simulink model "FTG"  (R2022a)
settings: Solver=ode4  StartTime=0.0  StopTime=100  FixedStep=0.01  RelTol=1e-3
PreLoadFcn:
  | listing = dir;
  | if (contains([listing .name], 'FLCC')) && (contains([listing .name], 'DYN'))
  |     addpath('./DYN', './FLCC', './FTG', './GPS', './INS', './MAP', './RALT', './TCAF');
  | elseif (contains([listing .name], 'FTG.slx'))
  |     addpath('../DYN', '../FLCC', '../FTG', '../GPS', '../INS', '../MAP', '../RALT', '../TCAF');
  | else
  | 
  | end
  | 
  | load('BUS_STRUCTURE_DYN.mat');
  | load('BUS_STRUCTURE_FLCC.mat');
  | load('BUS_STRUCTURE_RALT.mat');
  | load('BUS_STRUCTURE_INS.mat');
  | load('BUS_STRUCTURE_GPS.mat');
  | load('BUS_STRUCTURE_SENSOR_INPUT.mat');
  | load('BusStructureDTF.mat');
  | load('BusStructureGCAWS.mat');
  | FTG_initState;
  | 
  | % Random number seed
  | if ~exist('ranNumSeed', 'var')
  |     ranNumSeed = 2034;
  | end
InitFcn:
  | listing = dir;
  | if (contains([listing .name], 'FLCC')) && (contains([listing .name], 'DYN'))
  |     addpath('./DYN', './FLCC', './FTG', './GPS', './INS', './MAP', './RALT', './TCAF');
  | elseif (contains([listing .name], 'FTG.slx'))
  |     addpath('../DYN', '../FLCC', '../FTG', '../GPS', '../INS', '../MAP', '../RALT', '../TCAF');
  | else
  | 
  | end
  | 
  | load('BUS_STRUCTURE_DYN.mat');
  | load('BUS_STRUCTURE_FLCC.mat');
  | load('BUS_STRUCTURE_RALT.mat');
  | load('BUS_STRUCTURE_INS.mat');
  | load('BUS_STRUCTURE_GPS.mat');
  | load('BUS_STRUCTURE_SENSOR_INPUT.mat');
  | load('BusStructureDTF.mat');
  | load('BusStructureGCAWS.mat');
  | FTG_initState;
  | 
  | % Random number seed
  | if ~exist('ranNumSeed', 'var')
  |     ranNumSeed = 2034;
  | end
values from neighbouring files (symbols this model uses):
  initState = struct    [FTG_initState.m]
undefined symbols (not defined in the file or in its folder): GPS, INS, RALT
libraries: simulink_extras x8
settings Model: Creator=ASCL  LastModifiedBy=ASCL
settings DataIOCC: ExternalInput=FTGScenario.getElement('IN_STICK'), [], [],FTGScenario.getElement('IN_FLIGHT_CMD'), []  LoadExternalInput=on  SaveOutput=off  DSMLogging=off  SaveTime=off  ReturnWorkspaceOutputs=off
settings OptimizationCC: BlockReduction=off  DefaultParameterBehavior=Inlined  UseDivisionForNetSlopeComputation=on  GainParamInheritBuiltInType=on  UseFloatMulNetSlope=on  ExpressionFolding=off  PassReuseOutputArgsAs=Individual arguments  ZeroExternalMemoryAtStartup=off  ZeroInternalMemoryAtStartup=off  EfficientFloat2IntCast=on  LifeSpan=inf  OptimizeBlockOrder=speed  DifferentSizesBufferReuse=on  EfficientTunableParamExpr=on
settings DebuggingCC: SignalInfNanChecking=warning  ReadBeforeWriteMsg=EnableAllAsError  WriteAfterWriteMsg=EnableAllAsError  WriteAfterReadMsg=EnableAllAsError  IntegerOverflowMsg=error  ParameterTunabilityLossMsg=error  UniqueDataStoreMsg=error  AssertControl=DisableAll  NonBusSignalsTreatedAsBus=error  SFInvalidInputDataAccessInChartInitDiag=error  SFTransitionOutsideNaturalParentDiag=error  SFUnreachableExecutionPathDiag=error  SFUndirectedBroadcastEventsDiag=error  IntegerSaturationMsg=error
settings HardwareCC: ProdBitPerPointer=32  ProdBitPerSizeT=32  ProdBitPerPtrDiffT=32  ProdLargestAtomicInteger=Long  ProdLargestAtomicFloat=Double  ProdEndianess=BigEndian  ProdWordSize=32  ProdLongLongMode=on  ProdHWDeviceType=Freescale->MPC83xx
settings ModelReferenceCC: ModelReferenceNumInstancesAllowed=Single
settings SFSimCC: SimCustomHeaderCode="#include \"MAP.h\""  SimUserSources=MAP.c  SimUserLibraries=WS2_32.LIB  CompileTimeRecursionLimit=0  EnableRuntimeRecursion=off  MATLABDynamicMemAlloc=off
settings RTWCC: SystemTargetFile=ert.tlc  TemplateMakefile=ert_default_tmf  GenerateReport=on  RTWUseSimCustomCode=on  CustomHeaderCode="#include \"MAP.h\""  CustomSource=MAP.c  CustomLibrary=WS2_32.LIB  BuildConfiguration=Faster Runs  IncludeHyperlinkInReport=on  LaunchReport=on  GenerateTraceInfo=on  GenerateTraceReport=on  GenerateTraceReportSl=on  GenerateTraceReportSf=on  GenerateTraceReportEml=on  GenerateCodeMetricsReport=on
settings CodeAppCC: ForceParamTrailComments=on  IgnoreCustomStorageClasses=off  OperatorAnnotations=on  SimulinkDataObjDesc=on  SFDataObjDesc=on  MATLABFcnDesc=on  InsertBlockDesc=on  StateflowObjectComments=on  MATLABSourceComments=on  EnableCustomComments=on  InlinedPrmAccess=Macros  ReqsInCode=on
settings ERTTargetCC: TargetLangStandard=C99 (ISO)  UtilityFuncGeneration=Shared location  GenerateSampleERTMain=on  IncludeMdlTerminateFcn=off  CombineSignalStateStructs=on  SupportAbsoluteTime=off  SupportNonFinite=off  SupportVariableSizeSignals=on  ParenthesesLevel=Standards  CastingMode=Standards  GenerateSharedConstants=off  InlinedParameterPlacement=NonHierarchical  ERTCustomFileTemplate=example_file_process.tlc  RateTransitionBlockCode=Function  PreserveIfCondition=on  ConvertIfToSwitch=off  EnableSignedLeftShifts=off  EnableSignedRightShifts=off

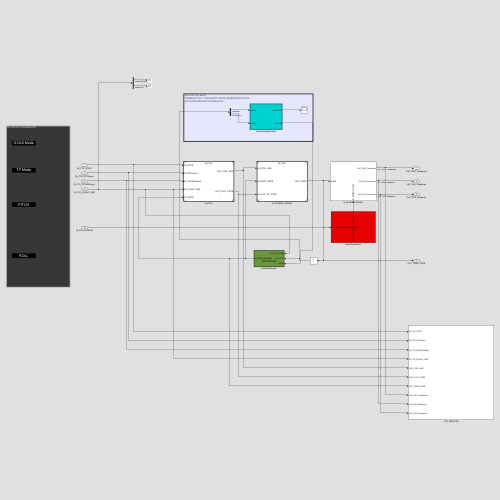
[thumbnail: Simulink's stored preview of the top-level diagram]
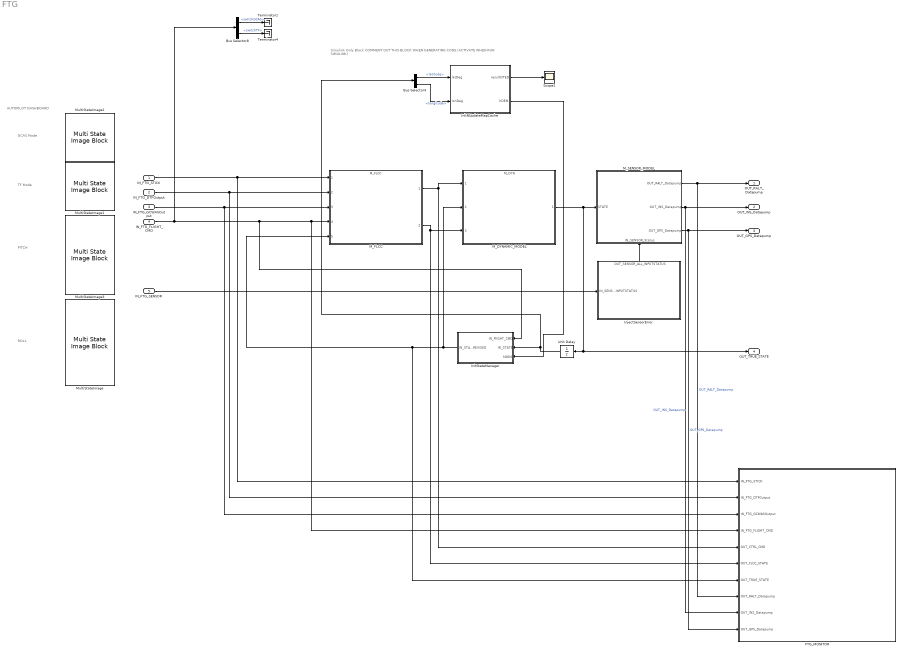
== system FTG ==
  note: GCAS Mode
  note: TF Mode
  note: AUTOPILOT DASHBOARD
  note: ROLL
  note: Simulink Only Block
      | COMMENT OUT THIS BLOCK WHEN GENERATING CODE
      | (ACTIVATE WHEN RUN SIMULINK)
  note: PITCH
  IN_FTG_STICK : Inport  OutDataTypeStr=Bus: BUS_FLCC_STICK  Interpolate=off  BusOutputAsStruct=on
  IN_FTG_DTFOutput : Inport  Port=2  OutDataTypeStr=Bus: DTFOutput  Interpolate=off  BusOutputAsStruct=on
  IN_FTG_GCWASOutput : Inport  Port=3  OutDataTypeStr=Bus: GCAWSOutput  Interpolate=off  BusOutputAsStruct=on
  IN_FTG_FLIGHT_CMD : Inport  Port=4  OutDataTypeStr=Bus: BUS_FLCC_FLIGHT_CMD  Interpolate=off  BusOutputAsStruct=on
  IN_FTG_SENSOR : Inport  Port=5  OutDataTypeStr=Bus: BUS_SENSOR_ALL_INPUTSTATUS  Interpolate=off  BusOutputAsStruct=on
  Bus Selector4 : BusSelector  OutputSignals=latitude,longitude
  Bus Selector8 : BusSelector  OutputSignals=switchGCAS,switchTF
  FTG_MONITOR : Subsystem
  InitNUpdateMapCache : Subsystem  TreatAsAtomicUnit=on
  InitStateManager : MATLAB Function  TreatAsAtomicUnit=on  SystemSampleTime=0.01
  InjectSensorError : Subsystem
      settings: PortSchema="{\"entries\":[{\"content\":{\"sides\":[{\"content\":{\"connectorIds\":[]},\"type\":\"ConnectorPlacement.EquallySpacedRectSide\",\"uuid\":\"6514be54-5250-42b1-89ec-96b3ca3204a4\"},{\"content\":{\"connectorIds\":[\"Out1\"],\"side\":\"RIGHT\"},\"type\":\"ConnectorPlacement.EquallySpacedRectSide\",\"uuid\":\"5a471b5b-ecab-4b12-91ae-851436c3af59\"},{\"content\":{\"connectorIds\":[\"In1\"],\"side\":\"TOP\"},\"type\":\"ConnectorPlacement.EquallySpacedRectSide\",\"uuid\":\"7b7a7584-bd38-4309-866b-d1039bf73b0c\"}]},\"type\":\"ConnectorPlacement.EquallySpacedConnector\",\"uuid\":\"354782b0-b839-451e-ba58-c4baa2a23659\"}],\"packageUris\":[\"http://schema.mathworks.com/mf0/Connector/R2020b\"],\"version\":\"1.0\"}"
  M_DYNAMIC_MODEL : ModelReference  ModelNameDialog=M_DYN.slx  SimulationMode=Normal  ModelReferenceVersion=1.350
  M_FLCC : ModelReference  ModelNameDialog=M_FLCC.slx  SimulationMode=Normal  ModelReferenceVersion=1.2865
  M_SENSOR_MODEL : Subsystem
      settings: PortSchema="{\"entries\":[{\"content\":{\"sides\":[{\"content\":{\"connectorIds\":[\"In1\"]},\"type\":\"ConnectorPlacement.EquallySpacedRectSide\",\"uuid\":\"880db95d-6046-467e-9f42-4d7f31e7d636\"},{\"content\":{\"connectorIds\":[\"Out1\",\"Out2\",\"Out3\"],\"side\":\"RIGHT\"},\"type\":\"ConnectorPlacement.EquallySpacedRectSide\",\"uuid\":\"4b6edf19-899b-47c2-bce1-8d6f85bc3049\"},{\"content\":{\"connectorIds\":[],\"side\":\"TOP\"},\"type\":\"ConnectorPlacement.EquallySpacedRectSide\",\"uuid\":\"fbda278b-8c92-4691-b142-226c9beb0c5e\"},{\"content\":{\"connectorIds\":[\"In2\"],\"side\":\"BOTTOM\"},\"type\":\"ConnectorPlacement.EquallySpacedRectSide\",\"uuid\":\"c82397e7-e882-4f57-bc38-1d7b6d57b901\"}]},\"type\":\"ConnectorPlacement.EquallySpacedConnector\",\"uuid\":\"2b9ff209-30b8-444e-97ac-554833487782\"}],\"packageUris\":[\"http://schema.mathworks.com/mf0/Connector/R2020b\"],\"version\":\"1.0\"}"
  MultiStateImage{,1..3} (4 alike) : MultiStateImageBlock
  Scope1 : Scope
  Terminator1 : Terminator
  Terminator4 : Terminator
  Unit Delay : UnitDelay  InitialCondition=initState  SampleTime=0.01  HasFrameUpgradeWarning=on
  OUT_RALT_Datapump : Outport  OutDataTypeStr=Bus: BUS_SENSOR_RALT_DP  SampleTime=0.01  BusOutputAsStruct=on
  OUT_INS_Datapump : Outport  Port=2  OutDataTypeStr=Bus: BUS_SENSOR_INS_DP  SampleTime=0.01  BusOutputAsStruct=on
  OUT_GPS_Datapump : Outport  Port=3  OutDataTypeStr=Bus: BUS_SENSOR_GPS_DP  SampleTime=0.01  BusOutputAsStruct=on
  OUT_TRUE_STATE : Outport  Port=4  OutDataTypeStr=Bus: BUS_DYN_STATE  SampleTime=0.01  BusOutputAsStruct=on
  wires:
  Bus Selector4/2 -> InitNUpdateMapCache/2(lonDeg)  "<longitude>"
  M_FLCC/2 -> M_DYNAMIC_MODEL/3, FTG_MONITOR/6(OUT_FLCC_STATE)
  IN_FTG_GCWASOutput/1 -> FTG_MONITOR/3(IN_FTG_GCWASOutput), M_FLCC/3
  M_SENSOR_MODEL/1(OUT_RALT_Datapump) -> OUT_RALT_Datapump/1, FTG_MONITOR/8(OUT_RALT_Datapump)  "OUT_RALT_Datapump"
  M_SENSOR_MODEL/3(OUT_GPS_Datapump) -> OUT_GPS_Datapump/1, FTG_MONITOR/10(OUT_GPS_Datapump)  "OUT_GPS_Datapump"
  IN_FTG_STICK/1 -> FTG_MONITOR/1(IN_FTG_STICK), M_FLCC/1
  IN_FTG_DTFOutput/1 -> FTG_MONITOR/2(IN_FTG_DTFOutput), M_FLCC/2
  Bus Selector4/1 -> InitNUpdateMapCache/1(latDeg)  "<latitude>"
  M_SENSOR_MODEL/2(OUT_INS_Datapump) -> OUT_INS_Datapump/1, FTG_MONITOR/9(OUT_INS_Datapump)  "OUT_INS_Datapump"
  M_FLCC/1 -> FTG_MONITOR/5(OUT_CTRL_CMD), M_DYNAMIC_MODEL/1
  M_DYNAMIC_MODEL/1 -> Unit Delay/1, OUT_TRUE_STATE/1, M_SENSOR_MODEL/1(STATE)
  Bus Selector8/2 -> Terminator4/1  "<switchTF>"
  Bus Selector8/1 -> Terminator1/1  "<switchGCAS>"
  InitNUpdateMapCache/1(resultDTED) -> Scope1/1
  IN_FTG_SENSOR/1 -> InjectSensorError/1(IN_SENSOR_ALL_INPUTSTATUS)
  InjectSensorError/1(OUT_SENSOR_ALL_INPUTSTATUS) -> M_SENSOR_MODEL/2(IN_SENSOR_Status)
  IN_FTG_FLIGHT_CMD/1 -> InitStateManager/1(IN_FlIGHT_CMD), FTG_MONITOR/4(IN_FTG_FLIGHT_CMD), M_FLCC/4, Bus Selector8/1
  InitStateManager/1(IN_STATE_REVISED) -> M_DYNAMIC_MODEL/2, FTG_MONITOR/7(OUT_TRUE_STATE), M_FLCC/5
  Unit Delay/1 -> InitStateManager/2(IN_STATE), Bus Selector4/1
  InitNUpdateMapCache/2(hDEM) -> InitStateManager/3(hDEM)

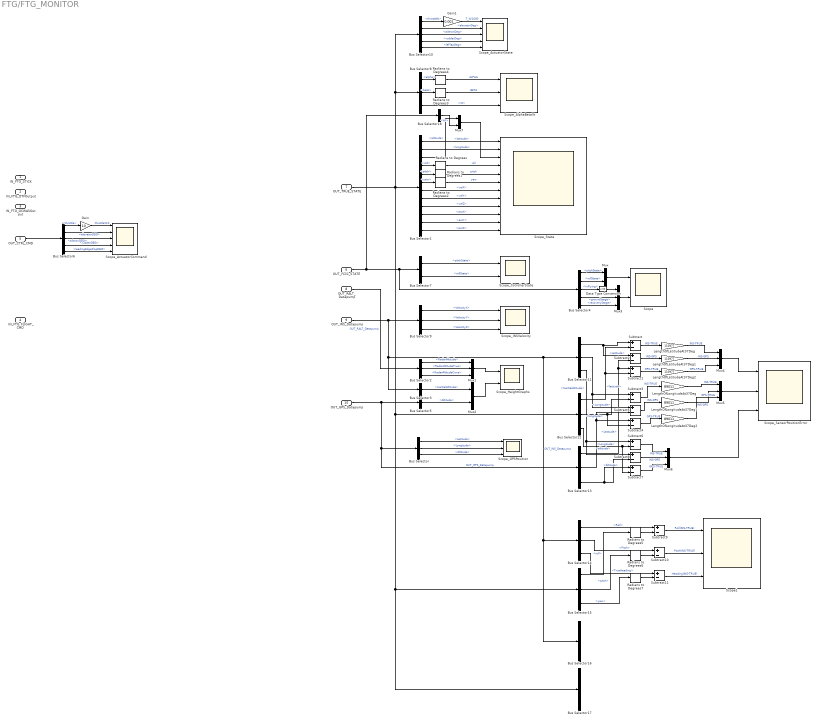
== system FTG/FTG_MONITOR ==
  IN_FTG_STICK : Inport
  IN_FTG_DTFOutput : Inport  Port=2
  IN_FTG_GCWASOutput : Inport  Port=3
  IN_FTG_FLIGHT_CMD : Inport  Port=4
  OUT_CTRL_CMD : Inport  Port=5
  OUT_FLCC_STATE : Inport  Port=6
  OUT_TRUE_STATE : Inport  Port=7
  OUT_RALT_Datapump : Inport  Port=8
  OUT_INS_Datapump : Inport  Port=9
  OUT_GPS_Datapump : Inport  Port=10
  Bus Selector : BusSelector  OutputSignals=Latitude,Longitude,Altitude
  Bus Selector1 : BusSelector  OutputSignals=latitude,longitude,altitude,roll,pitch,yaw,velX,velY,velZ,accX,accY,accZ
  Bus Selector10 : BusSelector  OutputSignals=throttleN,elevatorDeg,aileronDeg,rudderDeg,leFlapDeg
  Bus Selector11 : BusSelector  OutputSignals=Latitude,Longitude,InertialAltitude
  Bus Selector12 : BusSelector  OutputSignals=latitude,longitude,altitude
  Bus Selector13 : BusSelector  OutputSignals=Latitude,Longitude,Altitude
  Bus Selector14 : BusSelector  OutputSignals=Roll,Pitch,TrueHeading
  Bus Selector15 : BusSelector  OutputSignals=roll,pitch,yaw
  Bus Selector16 : BusSelector  OutputSignals=VelocityX,VelocityY,VelocityZ
  Bus Selector17 : BusSelector  OutputSignals=velX,velY,velZ
  Bus Selector18 : BusSelector  OutputSignals=h0
  Bus Selector2 : BusSelector  OutputSignals=RadarAltitude,RadarAltitudeTrue,RadarAltitudeCone
  Bus Selector3 : BusSelector  OutputSignals=InertialAltitude
  Bus Selector4 : BusSelector  OutputSignals=pitchState,rollState,inFlying,groundStage,recoveryStage
  Bus Selector5 : BusSelector  OutputSignals=Altitude
  Bus Selector6 : BusSelector  OutputSignals=throttle,elevatorDEG,aileronDEG,rudderDEG,leadingEdgeFlapDEG
  Bus Selector7 : BusSelector  OutputSignals=pitchState,rollState
  Bus Selector8 : BusSelector  OutputSignals=alpha,beta,Vt
  Bus Selector9 : BusSelector  OutputSignals=VelocityX,VelocityY,VelocityZ
  Data Type Conversion : DataTypeConversion  OutDataTypeStr=uint8  SaturateOnIntegerOverflow=off  RndMeth=Floor
  Gain : Gain  Gain=10
  Gain1 : Gain  Gain=0.001
  LengthOfLatitudeAt37Deg : Gain  Gain=110977
  LengthOfLatitudeAt37Deg1 : Gain  Gain=110977
  LengthOfLatitudeAt37Deg2 : Gain  Gain=110977
  LengthOfLongitudeAt37Deg : Gain  Gain=89011
  LengthOfLongitudeAt37Deg1 : Gain  Gain=89011
  LengthOfLongitudeAt37Deg2 : Gain  Gain=89011
  Mux : Mux  Inputs=2
  Mux{1,3..6} (5 alike) : Mux  Inputs=3
  Mux2 : Mux  Inputs=2
  Mux7 : Mux  Inputs=2
  Radians to Degrees{,1..7} (8 alike) : simulink_extras/Transformations/Radians to Degrees
  Scope : Scope  NumInputPorts=2
  Scope1 : Scope  NumInputPorts=3
  Scope_ActuatorCommand : Scope  NumInputPorts=5
  Scope_ActuatorState : Scope  NumInputPorts=5
  Scope_AlphaBetaVt : Scope  NumInputPorts=3
  Scope_CotrollerState : Scope  NumInputPorts=2
  Scope_GPSPosition : Scope  NumInputPorts=3
  Scope_HeightGraphs : Scope  NumInputPorts=2
  Scope_INSVelocity : Scope  NumInputPorts=3
  Scope_SensorPositionError : Scope  NumInputPorts=3
  Scope_State : Scope  NumInputPorts=12
  Subtract{,1..11} (12 alike) : Sum  Inputs=+-
  wires:
  Bus Selector1/9 -> Scope_State/9  "<velZ>"
  Bus Selector1/10 -> Scope_State/10  "<accX>"
  Bus Selector1/4 -> Radians to Degrees/1  "<roll>"
  Bus Selector1/1 -> Scope_State/1  "<latitude>"
  Radians to Degrees/1 -> Scope_State/4  "roll"
  Radians to Degrees1/1 -> Scope_State/5  "pitch"
  Bus Selector1/7 -> Scope_State/7  "<velX>"
  Bus Selector1/12 -> Scope_State/12  "<accZ>"
  Bus Selector1/2 -> Scope_State/2  "<longitude>"
  Bus Selector1/8 -> Scope_State/8  "<velY>"
  Bus Selector1/11 -> Scope_State/11  "<accY>"
  Bus Selector1/6 -> Radians to Degrees2/1  "<yaw>"
  Radians to Degrees2/1 -> Scope_State/6  "yaw"
  Bus Selector1/3 -> Mux7/1  "<altitude>"
  Bus Selector1/5 -> Radians to Degrees1/1  "<pitch>"
  Bus Selector9/1 -> Scope_INSVelocity/1  "<VelocityX>"
  Bus Selector9/3 -> Scope_INSVelocity/3  "<VelocityZ>"
  Bus Selector9/2 -> Scope_INSVelocity/2  "<VelocityY>"
  Bus Selector3/1 -> Mux2/1  "<InertialAltitude>"
  Bus Selector5/1 -> Mux2/2  "<Altitude>"
  Mux2/1 -> Scope_HeightGraphs/2
  Bus Selector2/3 -> Mux1/3  "<RadarAltitudeCone>"
  Bus Selector2/1 -> Mux1/1  "<RadarAltitude>"
  OUT_RALT_Datapump/1 -> Bus Selector2/1  "OUT_RALT_Datapump"
  OUT_INS_Datapump/1 -> Bus Selector3/1, Bus Selector16/1, Bus Selector14/1, Bus Selector11/1, Bus Selector9/1  "OUT_INS_Datapump"
  Mux1/1 -> Scope_HeightGraphs/1
  Bus Selector2/2 -> Mux1/2  "<RadarAltitudeTrue>"
  Bus Selector/2 -> Scope_GPSPosition/2  "<Longitude>"
  OUT_GPS_Datapump/1 -> Bus Selector13/1, Bus Selector/1, Bus Selector5/1  "OUT_GPS_Datapump"
  Bus Selector/3 -> Scope_GPSPosition/3  "<Altitude>"
  Bus Selector/1 -> Scope_GPSPosition/1  "<Latitude>"
  Bus Selector7/2 -> Scope_CotrollerState/2  "<rollState>"
  OUT_FLCC_STATE/1 -> Bus Selector18/1, Bus Selector4/1, Bus Selector7/1
  Bus Selector7/1 -> Scope_CotrollerState/1  "<pitchState>"
  Bus Selector6/2 -> Scope_ActuatorCommand/2  "<elevatorDEG>"
  OUT_CTRL_CMD/1 -> Bus Selector6/1
  Bus Selector6/4 -> Scope_ActuatorCommand/4  "<rudderDEG>"
  Bus Selector6/1 -> Gain/1  "<throttle>"
  Bus Selector6/3 -> Scope_ActuatorCommand/3  "<aileronDEG>"
  Bus Selector4/1 -> Mux/1  "<pitchState>"
  Bus Selector4/2 -> Mux/2  "<rollState>"
  Bus Selector4/3 -> Data Type Conversion/1  "<inFlying>"
  Bus Selector4/4 -> Mux3/2  "<groundStage>"
  Bus Selector4/5 -> Mux3/3  "<recoveryStage>"
  Mux/1 -> Scope/1
  Mux3/1 -> Scope/2
  Data Type Conversion/1 -> Mux3/1
  Bus Selector8/1 -> Radians to Degrees4/1  "<alpha>"
  Bus Selector8/2 -> Radians to Degrees3/1  "<beta>"
  Radians to Degrees4/1 -> Scope_AlphaBetaVt/1  "ALPHA"
  Radians to Degrees3/1 -> Scope_AlphaBetaVt/2  "BETA"
  Bus Selector8/3 -> Scope_AlphaBetaVt/3  "<Vt>"
  Gain/1 -> Scope_ActuatorCommand/1  "throttleX10"
  Bus Selector6/5 -> Scope_ActuatorCommand/5  "<leadingEdgeFlapDEG>"
  Bus Selector10/1 -> Gain1/1  "<throttleN>"
  Bus Selector10/5 -> Scope_ActuatorState/5  "<leFlapDeg>"
  Bus Selector10/4 -> Scope_ActuatorState/4  "<rudderDeg>"
  Bus Selector10/3 -> Scope_ActuatorState/3  "<aileronDeg>"
  Bus Selector10/2 -> Scope_ActuatorState/2  "<elevatorDeg>"
  Gain1/1 -> Scope_ActuatorState/1  "T_N/1000"
  Bus Selector11/1 -> Subtract2/1, Subtract/1  "<Latitude>"
  Bus Selector12/1 -> Subtract1/2, Subtract/2  "<latitude>"
  LengthOfLatitudeAt37Deg/1 -> Mux4/1  "INS-TRUE"
  Bus Selector13/1 -> Subtract1/1, Subtract2/2  "<Latitude>"
  Subtract2/1 -> LengthOfLatitudeAt37Deg1/1  "INS-GPS"
  LengthOfLongitudeAt37Deg2/1 -> Mux5/3  "GPS-TRUE"
  LengthOfLongitudeAt37Deg1/1 -> Mux5/2  "INS-GPS"
  LengthOfLongitudeAt37Deg/1 -> Mux5/1  "INS-TRUE"
  Subtract6/1 -> Mux6/1  "INS-TRUE"
  Subtract8/1 -> Mux6/2  "INS-GPS"
  Subtract7/1 -> Mux6/3  "GPS-TRUE"
  Mux6/1 -> Scope_SensorPositionError/3
  Bus Selector11/2 -> Subtract5/1, Subtract3/1  "<Longitude>"
  Bus Selector12/2 -> Subtract4/2, Subtract3/2  "<longitude>"
  Bus Selector13/2 -> Subtract4/1, Subtract5/2  "<Longitude>"
  Bus Selector11/3 -> Subtract8/1, Subtract6/1  "<InertialAltitude>"
  Bus Selector13/3 -> Subtract7/1, Subtract8/2  "<Altitude>"
  Bus Selector12/3 -> Subtract7/2, Subtract6/2  "<altitude>"
  Mux4/1 -> Scope_SensorPositionError/1
  Mux5/1 -> Scope_SensorPositionError/2
  Subtract/1 -> LengthOfLatitudeAt37Deg/1  "INS-TRUE"
  LengthOfLatitudeAt37Deg1/1 -> Mux4/2  "INS-GPS"
  LengthOfLatitudeAt37Deg2/1 -> Mux4/3  "GPS-TRUE"
  Subtract1/1 -> LengthOfLatitudeAt37Deg2/1  "GPS-TRUE"
  Subtract3/1 -> LengthOfLongitudeAt37Deg/1  "INS-TRUE"
  Subtract5/1 -> LengthOfLongitudeAt37Deg1/1  "INS-GPS"
  Subtract4/1 -> LengthOfLongitudeAt37Deg2/1  "GPS-TRUE"
  Bus Selector14/1 -> Subtract9/1  "<Roll>"
  Bus Selector14/2 -> Subtract10/1  "<Pitch>"
  Bus Selector14/3 -> Subtract11/1  "<TrueHeading>"
  Bus Selector15/1 -> Radians to Degrees5/1  "<roll>"
  Bus Selector15/2 -> Radians to Degrees6/1  "<pitch>"
  Bus Selector15/3 -> Radians to Degrees7/1  "<yaw>"
  Subtract10/1 -> Scope1/2  "Pitch(INS-TRUE)"
  Subtract9/1 -> Scope1/1  "Roll(INS-TRUE)"
  Subtract11/1 -> Scope1/3  "Heading(INS-TRUE)"
  OUT_TRUE_STATE/1 -> Bus Selector17/1, Bus Selector15/1, Bus Selector12/1, Bus Selector10/1, Bus Selector8/1, Bus Selector1/1
  Radians to Degrees5/1 -> Subtract9/2
  Radians to Degrees6/1 -> Subtract10/2
  Radians to Degrees7/1 -> Subtract11/2
  Bus Selector18/1 -> Mux7/2  "<h0>"
  Mux7/1 -> Scope_State/3

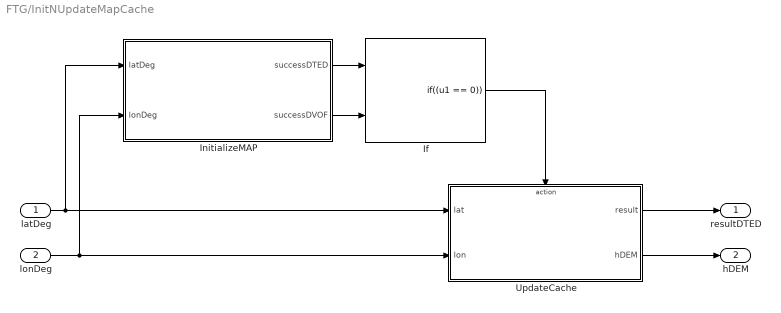
== system FTG/InitNUpdateMapCache ==
  latDeg : Inport  OutDataTypeStr=double
  lonDeg : Inport  Port=2  OutDataTypeStr=double
  If : If  NumInputs=2  IfExpression=(u1 == 0)  ShowElse=off
  InitializeMAP : MATLAB Function  TreatAsAtomicUnit=on  SystemSampleTime=0.01
  UpdateCache : Subsystem  TreatAsAtomicUnit=on
  resultDTED : Outport  VectorParamsAs1DForOutWhenUnconnected=off
  hDEM : Outport  Port=2
  wires:
  lonDeg/1 -> InitializeMAP/2(lonDeg), UpdateCache/2(lon)
  UpdateCache/1(result) -> resultDTED/1
  InitializeMAP/1(successDTED) -> If/1
  latDeg/1 -> InitializeMAP/1(latDeg), UpdateCache/1(lat)
  InitializeMAP/2(successDVOF) -> If/2
  If/1 -> UpdateCache/Action
  UpdateCache/2(hDEM) -> hDEM/1

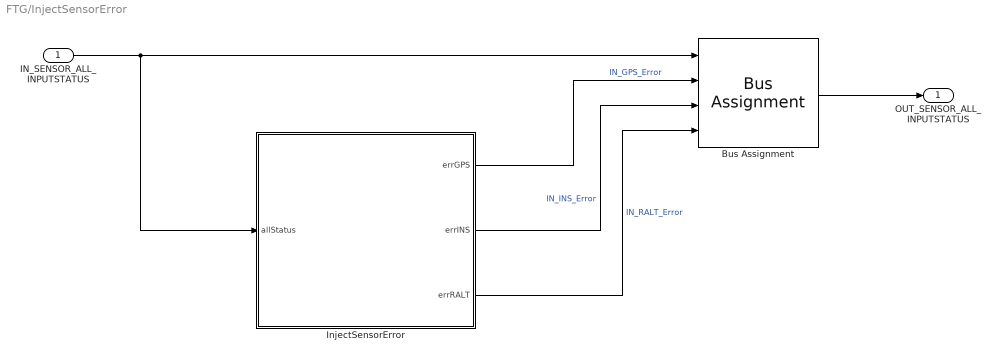
== system FTG/InjectSensorError ==
  IN_SENSOR_ALL_INPUTSTATUS : Inport  OutDataTypeStr=Bus: BUS_SENSOR_ALL_INPUTSTATUS
  Bus Assignment : BusAssignment  AssignedSignals=GPS.InjectedError,INS.InjectedError,RALT.InjectedError
  InjectSensorError : MATLAB Function  TreatAsAtomicUnit=on  SystemSampleTime=0.01
      settings: RTWSystemCode=Nonreusable function  RTWFcnNameOpts=Use subsystem name  RTWFileNameOpts=Use subsystem name
  OUT_SENSOR_ALL_INPUTSTATUS : Outport  OutDataTypeStr=Bus: BUS_SENSOR_ALL_INPUTSTATUS
  wires:
  InjectSensorError/2(errINS) -> Bus Assignment/3  "IN_INS_Error"
  InjectSensorError/1(errGPS) -> Bus Assignment/2  "IN_GPS_Error"
  InjectSensorError/3(errRALT) -> Bus Assignment/4  "IN_RALT_Error"
  IN_SENSOR_ALL_INPUTSTATUS/1 -> InjectSensorError/1(allStatus), Bus Assignment/1
  Bus Assignment/1 -> OUT_SENSOR_ALL_INPUTSTATUS/1

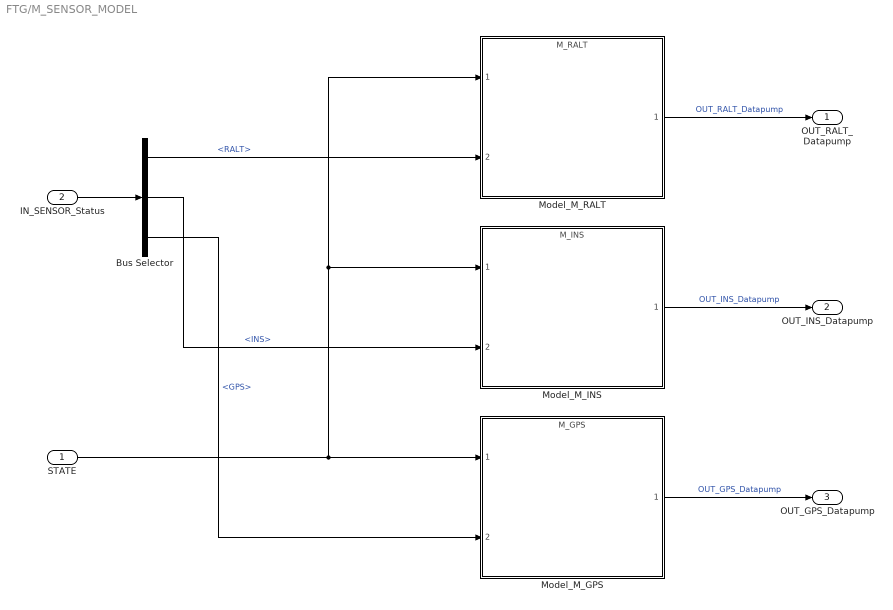
== system FTG/M_SENSOR_MODEL ==
  STATE : Inport  OutDataTypeStr=Bus: BUS_DYN_STATE
  IN_SENSOR_Status : Inport  Port=2  OutDataTypeStr=Bus: BUS_SENSOR_ALL_INPUTSTATUS
  Bus Selector : BusSelector  OutputSignals=RALT,INS,GPS
  Model_M_GPS : ModelReference  ModelNameDialog=M_GPS.slx  SimulationMode=Normal  ModelReferenceVersion=1.230
  Model_M_INS : ModelReference  ModelNameDialog=M_INS.slx  SimulationMode=Normal  ModelReferenceVersion=1.622
  Model_M_RALT : ModelReference  ModelNameDialog=M_RALT.slx  SimulationMode=Normal  ModelReferenceVersion=1.541
  OUT_RALT_Datapump : Outport  OutDataTypeStr=Bus: BUS_SENSOR_RALT_DP
  OUT_INS_Datapump : Outport  Port=2  OutDataTypeStr=Bus: BUS_SENSOR_INS_DP
  OUT_GPS_Datapump : Outport  Port=3  OutDataTypeStr=Bus: BUS_SENSOR_GPS_DP
  wires:
  STATE/1 -> Model_M_RALT/1, Model_M_INS/1, Model_M_GPS/1
  Model_M_RALT/1 -> OUT_RALT_Datapump/1  "OUT_RALT_Datapump"
  Model_M_INS/1 -> OUT_INS_Datapump/1  "OUT_INS_Datapump"
  Model_M_GPS/1 -> OUT_GPS_Datapump/1  "OUT_GPS_Datapump"
  Bus Selector/3 -> Model_M_GPS/2  "<GPS>"
  Bus Selector/2 -> Model_M_INS/2  "<INS>"
  Bus Selector/1 -> Model_M_RALT/2  "<RALT>"
  IN_SENSOR_Status/1 -> Bus Selector/1

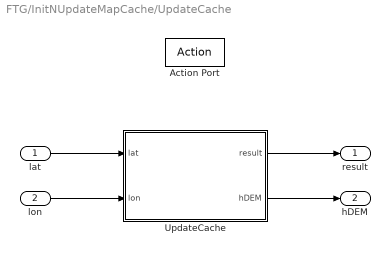
== system FTG/InitNUpdateMapCache/UpdateCache ==
  lat : Inport
  lon : Inport  Port=2
  Action Port : ActionPort  ActionPortLabel=if((u1 == 0))
  UpdateCache : MATLAB Function  TreatAsAtomicUnit=on  SystemSampleTime=0.01
  result : Outport  VectorParamsAs1DForOutWhenUnconnected=off
  hDEM : Outport  Port=2
  wires:
  UpdateCache/1(result) -> result/1
  lat/1 -> UpdateCache/1(lat)
  lon/1 -> UpdateCache/2(lon)
  UpdateCache/2(hDEM) -> hDEM/1

== matlab function FTG/InitStateManager ==
  data: IN_FlIGHT_CMD input Bus: BUS_FLCC_FLIGHT_CMD; IN_STATE input Bus: BUS_DYN_STATE; IN_STATE_REVISED output Bus: BUS_DYN_STATE; hDEM input
function IN_STATE_REVISED = InitStateManager(IN_FlIGHT_CMD, IN_STATE, hDEM)
%InitStateManager 비행모드, initState, Ground 모드를 고려하여 초기 상태값을
% 초기화한다. Ground 모드로 비행시 항공기 상태를 GROUND IDLE 상태로 초기화
% 한다. [RPY -> C_b_n], [velXYZ -> velNED], [(~) -> alpha, beta, Vt] 
persistent firstRun
if isempty(firstRun)
    firstRun = true;
end


IN_STATE_REVISED = IN_STATE;

if (firstRun)

    h0 = hDEM;

    if ( (IN_FlIGHT_CMD.flightMode == uint8(2)) || (IN_FlIGHT_CMD.flightMode == uint8(3)) )

        IN_STATE_REVISED.altitude = h0;
        IN_STATE_REVISED.roll = 0.0;
        IN_STATE_REVISED.pitch = 0.0;
        IN_STATE_REVISED.velN = 0.0;
        IN_STATE_REVISED.velE = 0.0;
        IN_STATE_REVISED.velD = 0.0;
        IN_STATE_REVISED.velX = 0.0;
        IN_STATE_REVISED.velY = 0.0;
        IN_STATE_REVISED.velZ = 0.0;
        IN_STATE_REVISED.omX = 0.0;
        IN_STATE_REVISED.omY = 0.0;
        IN_STATE_REVISED.omZ = 0.0;
        IN_STATE_REVISED.accX = 0.0;
        IN_STATE_REVISED.accY = 0.0;
        IN_STATE_REVISED.accZ = 0.0;
        IN_STATE_REVISED.omDotX = 0.0;
        IN_STATE_REVISED.omDotY = 0.0;
        IN_STATE_REVISED.omDotZ = 0.0;
        IN_STATE_REVISED.elevatorDeg = 0.0;
        IN_STATE_REVISED.aileronDeg = 0.0;
        IN_STATE_REVISED.rudderDeg = 0.0;
        IN_STATE_REVISED.leFlapDeg = 0.0;
        IN_STATE_REVISED.timeTag = uint16(0);
        IN_STATE_REVISED.groundStage = uint8(0);    
        IN_STATE_REVISED.wow = true;
        IN_STATE_REVISED.f_ib_b = [0; 0; 9.8];

        cRol = cos(IN_STATE_REVISED.roll);
        sRol = sin(IN_STATE_REVISED.roll);
        cPit = cos(IN_STATE_REVISED.pitch);
        sPit = sin(IN_STATE_REVISED.pitch);
        cYaw = cos(IN_STATE_REVISED.yaw);
        sYaw = sin(IN_STATE_REVISED.yaw);
        IN_STATE_REVISED.C_b_n = ...
            [ cPit*cYaw, sRol*sPit*cYaw-cRol*sYaw, cRol*sPit*cYaw+sRol*sYaw;...
            cPit*sYaw, sRol*sPit*sYaw+cRol*cYaw, cRol*sPit*sYaw-sRol*cYaw;...
            -sPit,                sRol*cPit,                cRol*cPit];

    end


    % Calculate (DCM) rotation matirx
    % Define trigonometric functions
    cRol = cos(IN_STATE_REVISED.roll);
    sRol = sin(IN_STATE_REVISED.roll);
    cPit = cos(IN_STATE_REVISED.pitch);
    sPit = sin(IN_STATE_REVISED.pitch);
    cYaw = cos(IN_STATE_REVISED.yaw);
    sYaw = sin(IN_STATE_REVISED.yaw);
    IN_STATE_REVISED.C_b_n = ...
        [ cPit*cYaw, sRol*sPit*cYaw-cRol*sYaw, cRol*sPit*cYaw+sRol*sYaw;...
        cPit*sYaw, sRol*sPit*sYaw+cRol*cYaw, cRol*sPit*sYaw-sRol*cYaw;...
        -sPit,                sRol*cPit,                cRol*cPit];

    % Calculate NED velocity
    velNED = zeros(3,1);
    velNED = IN_STATE_REVISED.C_b_n ... 
        * [IN_STATE_REVISED.velX; IN_STATE_REVISED.velY; IN_STATE_REVISED.velZ];
    IN_STATE_REVISED.velN = velNED(1);
    IN_STATE_REVISED.velE = velNED(2);
    IN_STATE_REVISED.velD = velNED(3);

    % Calculate alpha, beta, Vt
    alpha = 0.0;
    beta = 0.0;
    TAS = 0.0;
    windVelNED = [IN_STATE_REVISED.windVelN; IN_STATE_REVISED.windVelE; IN_STATE_REVISED.windVelD];
    [alpha, beta, TAS] = GetKinematicVariables(IN_STATE_REVISED.C_b_n, velNED, windVelNED);
    IN_STATE_REVISED.alpha = alpha;
    IN_STATE_REVISED.beta = beta;
    IN_STATE_REVISED.Vt = TAS;
    IN_STATE_REVISED.f_ib_b = [0; 0; 9.8];

    firstRun = false;
    
else

end

end

function [alpha, beta, TAS] = GetKinematicVariables(C_b_n, velNED, windVelNED)
%GetKinematicVariables

% Initialize
alpha   = 0.0;
beta    = 0.0;
TAS     = 0.0;

% Body to NED
% cRol = cos(attiEuler(1));
% sRol = sin(attiEuler(1));
% cPit = cos(attiEuler(2));
% sPit = sin(attiEuler(2));
% cYaw = cos(attiEuler(3));
% sYaw = sin(attiEuler(3));

% Coordinate Transformation
% NED to Body
C_n_b = C_b_n';
% C_n_b   = [              cPit*cYaw,                cPit*sYaw,     -sPit;...
%           sRol*sPit*cYaw-cRol*sYaw, sRol*sPit*sYaw+cRol*cYaw, sRol*cPit;...
%           cRol*sPit*cYaw+sRol*sYaw, cRol*sPit*sYaw-sRol*cYaw, cRol*cPit];

% Velocity relative to the wind
vRA_n = [velNED(1) - windVelNED(1); ...
    velNED(2) - windVelNED(2); ...
    velNED(3) - windVelNED(3)];
vRA_b = C_n_b * vRA_n;

TAS = norm(vRA_n);

% AOA
if (norm(vRA_b) < 0.5)
    alpha = 0.0;
else
    alpha = atan2(vRA_b(3), vRA_b(1));
end

% Sideslip Angle
if ( (abs(vRA_b(2)) < TAS) && (TAS > 0.5) )
    beta    = asin(vRA_b(2) / TAS);
else
    % Abnormal case
    beta    = 0.0;
end
end

== matlab function FTG/InjectSensorError/InjectSensorError ==
  data: errGPS output; errINS output; errRALT output; allStatus input Bus: BUS_SENSOR_ALL_INPUTSTATUS
function [errGPS, errINS, errRALT] = InjectSensorError(allStatus)
%InjectSensorError
% Output
% - errRALT: heightAGL(1) (m)
% - errINS : [llh(3), velXYZ(3), euler(3), accXYZ(3)]
%             ddm     mps        rad       mps2
% - errGPS : [llh(3), velNED(3)]
%             ddm     mps
persistent time dt
if isempty(time)
    time = 0.0;
end
if isempty(dt)
    dt = 0.01;
end

% GPS
errGPS = zeros(6, 1);
if (allStatus.GPS.InputActivated)
    errGPS = allStatus.GPS.InjectedError;
else
    errGPS = zeros(6, 1);
end
% errGPS = getLLHBias(errGPS, [0.01, 0.01, 500], time, 10, 1);
% errGPS = getLLHBias(errGPS, [-0.01, 0.01, 500], time, 20, 1);
% errGPS = getLLHBias(errGPS, [-0.02, -0.02, -500], time, 30, 1);
% errGPS = getLLHBias(errGPS, [0.01, -0.05, 500], time, 40, 1);
% errGPS = getVelBias(errGPS, [10, 10, 10], time, 50, 1);

% INS
errINS = zeros(12, 1);
if (allStatus.INS.InputActivated)
    errINS = allStatus.INS.InjectedError;
else
    errINS = zeros(12, 1);
end
% errINS = getLLHBias(errINS, [0.001, 0.001, 10], time, 0, inf);
% errINS = getLLHBias(errINS, [0.03, -0.04, 10], time, 20, 1);
% errINS = getLLHBias(errINS, [-0.02, 0.04, 20], time, 30, 0.08);
% errINS = getLLHBias(errINS, [0.02, 0.04, 10], time, 40, 0.04);
% errINS = getLLHBias(errINS, [-0.02, -0.04, 10], time, 50, 0.04);

% RALT
errRALT = 0.0;
if (allStatus.RALT.InputActivated)
    errRALT = allStatus.RALT.InjectedError;
else
    errRALT = 0.0;
end
% errRALT = getRALTBias(errRALT, 800, time, 10, 0.08);
% errRALT = getRALTBias(errRALT, 300, time, 20, 0.08);
% errRALT = getRALTBias(errRALT, -400, time, 30, 0.08);
% errRALT = getRALTBias(errRALT, 600, time, 40, 0.08);
% errRALT = getRALTBias(errRALT, -300, time, 50, 0.08);

time = time + dt;

end

%% Internal Functions
function err = getLLHBias(err, errValues, curTime, triggerTime, duration)
    if (triggerTime <= curTime) && (curTime <= triggerTime+duration)
        err(1) = errValues(1);
        err(2) = errValues(2);
        err(3) = errValues(3);
    else
    end
    
end

function err = getVelBias(err, errValues, curTime, triggerTime, duration)
    if (triggerTime <= curTime) && (curTime <= triggerTime+duration)
        err(4) = errValues(1);
        err(5) = errValues(2);
        err(6) = errValues(3);
    else
    end
    
end

function err = getRALTBias(err, errValues, curTime, triggerTime, duration)
    if (triggerTime <= curTime) && (curTime <= triggerTime+duration)
        err = errValues;
    else
    end
end

== matlab function FTG/InitNUpdateMapCache/InitializeMAP ==
  data: successDTED output; successDVOF output; latDeg input; lonDeg input
function [successDTED, successDVOF] = InitializeMAP(latDeg, lonDeg)
%InitializeMAP

% Persistent variable
persistent firstRun
if isempty(firstRun)
    firstRun = true;
end

% Initialize output
flagDTED = int32(1);
flagDVOF = int32(1);
successDTED = int32(1);
successDVOF = int32(1);
hDEM = 0.0;

if firstRun
    % Path of DTED data
    pathDTED = 'C:\Users\ASCL\Documents\GitHub\DTNS\MAP\MAP_DB';

    % Length of DETD data path
    strLenDTED = int32(strlength(pathDTED));
    
    hDEM = coder.ceval('MAPGetTerrainHeight', latDeg, lonDeg);
    if IsNear(hDEM, -1.0)
        % Call [ InitialMap ] : 맵 폴더 위치 설정
        flagDTED = coder.ceval('InitialMap', pathDTED, strLenDTED );
        successDTED = flagDTED;
        if (~successDTED)
            firstRun = false;
        end
    else
        successDTED = int32(0);
        firstRun = false;       
    end
else
    successDTED = int32(0);
    successDVOF = int32(0);
end

== matlab function FTG/InitNUpdateMapCache/UpdateCache/UpdateCache ==
  data: result output; lat input; lon input; hDEM output
function [result, hDEM] = UpdateCache(lat, lon)
%UpdateCache

% Persistent variables
persistent latPrev lonPrev
if isempty(latPrev)
    latPrev = 0.0;
end
if isempty(lonPrev)
    lonPrev = 0.0;
end

hDEM = 0.0;

% Initialize output
result = int32(1);

if ( abs(lat - latPrev) > 0.05 ) || ( abs(lon - lonPrev) > 0.05)
    result = coder.ceval('UpdateCache', lat, lon);
    hDEM = coder.ceval('MAPGetTerrainHeight', lat, lon);

    if result == 0
        latPrev = lat;
        lonPrev = lon;
    end
else
    hDEM = coder.ceval('MAPGetTerrainHeight', lat, lon);
end
